simulink model "RR_1DOF"  (R2023b)
settings: Solver=VariableStepAuto  StartTime=0.0  StopTime=1200  RelTol=1e-3
values from neighbouring files (symbols this model uses):
  G = 32.174    [RR.mat]
  RR_AERO_S = 8.85    [RR.mat]
  RR_Fuel_Consumption = [7.65146967075e-05 0.000426716577792]    [RR.mat]
  RR_Fuel_Mass = 0.422701560266    [RR.mat]
  RR_Fuel_Volume = 0.267361092544    [RR.mat]
  RR_Motors_Thrust = [4.04656097579 98.9159349639]    [RR.mat]
  RR_Motors_Thrust_Alt_Lut = [0 10000 20000 30000]    [RR.mat]
  RR_Motors_Thrust_Pct_Lut = [1 0.705882352941 0.470588235294 0.352941176471]    [RR.mat]
  RR_PD_ALT = [0 10000 30000]    [RR.mat]
  RR_PD_CD = [0.03954  0.0426  0.05073; 0.01481  0.01557  0.0175; 0.0113  0.01182  0.01313; 0.0103  0.01077  0.01191]    [RR.mat]
  RR_PD_MACH = [0.001 0.1 0.5 0.9]    [RR.mat]
  RR_Total_Dry_Mass = 1.55129843973    [RR.mat]
undefined symbols (not defined in the file or in its folder): magnitude
libraries: aerolibatmos2 x1, aerolibasang x1, simulink x1
settings Model: Creator=jrighetti  LastModifiedBy=jrighetti

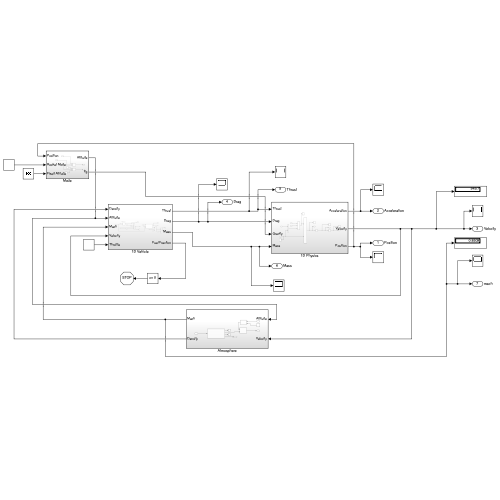
[thumbnail: Simulink's stored preview of the top-level diagram]
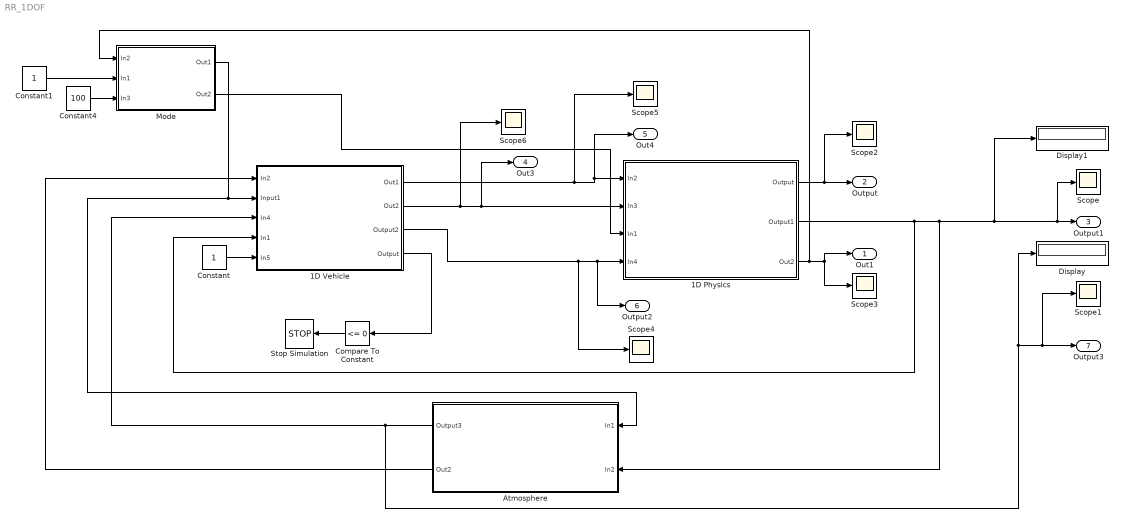
== system RR_1DOF ==
  1D Physics : Subsystem
  1D Vehicle : Subsystem
  Atmosphere : Subsystem
  Compare To Constant : simulink/Logic and Bit Operations/Compare To Constant  relop=<=  const=0  OutDataTypeStr=boolean
  Constant : Constant
  Constant1 : Constant
  Constant4 : Constant  Value=100
  Display : Display
  Display1 : Display
  Mode : Subsystem
  Scope{,1..6} (7 alike) : Scope
  Stop Simulation : Stop
  Out1 : Outport  SignalName=Position
  Output : Outport  Port=2  SignalName=Acceleration
  Output1 : Outport  Port=3  SignalName=Velocity
  Out3 : Outport  Port=4  SignalName=Drag
  Out4 : Outport  Port=5  SignalName=Thrust
  Output2 : Outport  Port=6  SignalName=Mass
  Output3 : Outport  Port=7  SignalName=mach
  wires:
  1D Vehicle/1(Out1) -> Scope5/1, Out4/1, 1D Physics/1(In2)
  1D Vehicle/2(Out2) -> Scope6/1, 1D Physics/2(In3), Out3/1
  1D Vehicle/4(Output) -> Compare To Constant/1
  1D Vehicle/3(Output2) -> Scope4/1, Output2/1, 1D Physics/4(In4)
  Constant/1 -> 1D Vehicle/5(In5)
  Atmosphere/1(Output3) -> Display/1, Scope1/1, Output3/1, 1D Vehicle/3(In4)
  1D Physics/1(Output) -> Scope2/1, Output/1
  1D Physics/3(Out2) -> Mode/1(In2), Out1/1, Scope3/1
  1D Physics/2(Output1) -> Atmosphere/2(In2), Display1/1, Scope/1, Output1/1, 1D Vehicle/4(In1)
  Compare To Constant/1 -> Stop Simulation/1
  Atmosphere/2(Out2) -> 1D Vehicle/1(In2)
  Constant4/1 -> Mode/3(In3)
  Mode/2(Out2) -> 1D Physics/3(In1)
  Constant1/1 -> Mode/2(In1)
  Mode/1(Out1) -> 1D Vehicle/2(Input1), Atmosphere/1(In1)

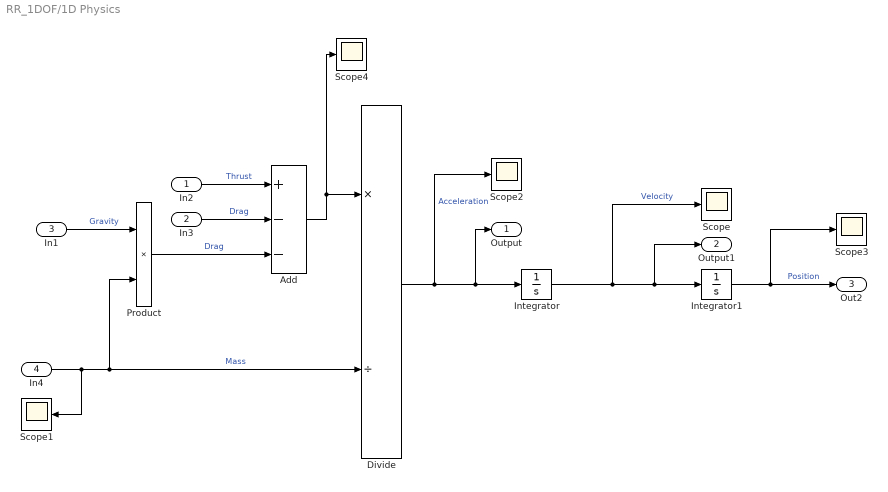
== system RR_1DOF/1D Physics ==
  In2 : Inport
  In3 : Inport  Port=2
  In1 : Inport  Port=3
  In4 : Inport  Port=4
  Add : Sum  Inputs=+--
  Divide : Product  Inputs=*/
  Integrator : Integrator
  Integrator1 : Integrator
  Product : Product
  Scope{,1..4} (5 alike) : Scope
  Output : Outport
  Output1 : Outport  Port=2
  Out2 : Outport  Port=3
  wires:
  Integrator1/1 -> Scope3/1, Out2/1  "Position"
  Add/1 -> Scope4/1, Divide/1
  Integrator/1 -> Integrator1/1, Output1/1, Scope/1  "Velocity"
  Divide/1 -> Scope2/1, Output/1, Integrator/1  "Acceleration"
  In2/1 -> Add/1  "Thrust"
  In3/1 -> Add/2  "Drag"
  In4/1 -> Scope1/1, Divide/2, Product/2  "Mass"
  In1/1 -> Product/1  "Gravity"
  Product/1 -> Add/3  "Drag"

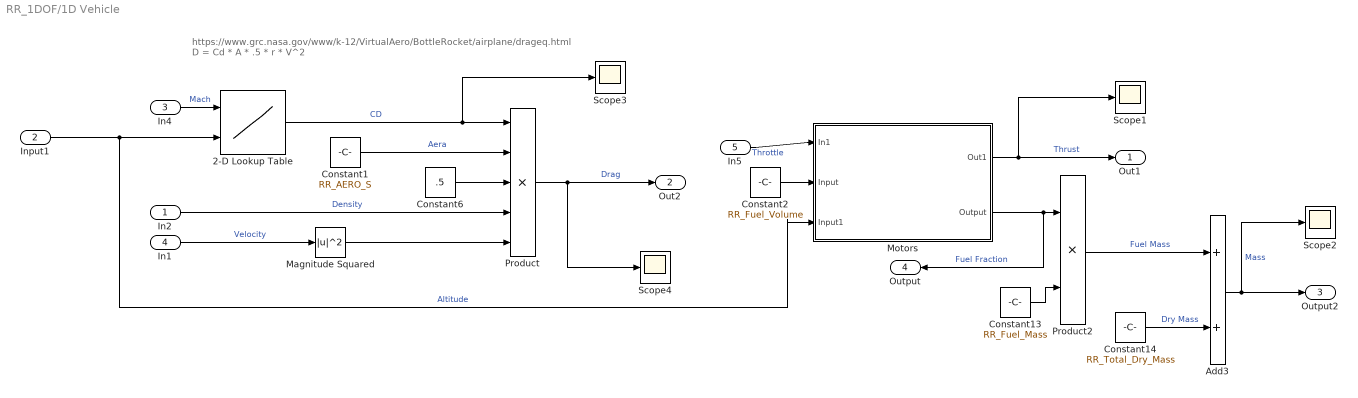
== system RR_1DOF/1D Vehicle ==
  note: https://www.grc.nasa.gov/www/k-12/VirtualAero/BottleRocket/airplane/drageq.html
      |
      | D = Cd * A * .5 * r * V^2
  In2 : Inport
  Input1 : Inport  Port=2
  In4 : Inport  Port=3
  In1 : Inport  Port=4
  In5 : Inport  Port=5
  2-D Lookup Table : Lookup_n-D  BreakpointsForDimension1=RR_PD_MACH  BreakpointsForDimension2=RR_PD_ALT  Table=RR_PD_CD  InternalRulePriority=Speed  RndMeth=Simplest
      settings: InputPortMap=u0,u1
  Add3 : Sum
  Constant1 : Constant  Value=RR_AERO_S
  Constant13 : Constant  Value=RR_Fuel_Mass
  Constant14 : Constant  Value=RR_Total_Dry_Mass
  Constant2 : Constant  Value=RR_Fuel_Volume
  Constant6 : Constant  Value=.5
  Magnitude Squared : Math  Operator=magnitude^2
  Motors : Subsystem
  Product : Product  Inputs=5
  Product2 : Product
  Scope{1..4} (4 alike) : Scope
  Out1 : Outport
  Out2 : Outport  Port=2
  Output2 : Outport  Port=3
  Output : Outport  Port=4
  wires:
  2-D Lookup Table/1 -> Scope3/1, Product/1  "CD"
  Motors/1(Out1) -> Scope1/1, Out1/1  "Thrust"
  Product/1 -> Scope4/1, Out2/1  "Drag"
  Constant1/1 -> Product/2  "Aera"
  Constant6/1 -> Product/3
  In2/1 -> Product/4  "Density"
  Magnitude Squared/1 -> Product/5
  In1/1 -> Magnitude Squared/1  "Velocity"
  Input1/1 -> Motors/3(Input1), 2-D Lookup Table/2  "Altitude"
  In4/1 -> 2-D Lookup Table/1  "Mach"
  Constant2/1 -> Motors/2(Input)
  Constant14/1 -> Add3/2  "Dry Mass"
  Motors/2(Output) -> Product2/1, Output/1  "Fuel Fraction"
  Constant13/1 -> Product2/2
  Product2/1 -> Add3/1  "Fuel Mass"
  Add3/1 -> Scope2/1, Output2/1  "Mass"
  In5/1 -> Motors/1(In1)  "Throttle"

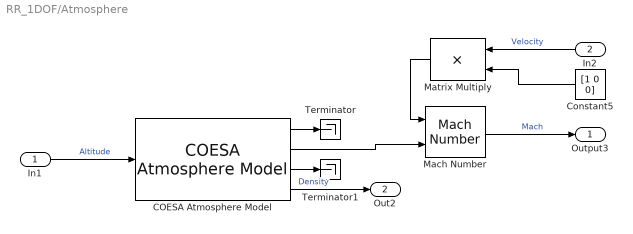
== system RR_1DOF/Atmosphere ==
  In1 : Inport
  In2 : Inport  Port=2
  COESA Atmosphere Model : aerolibatmos2/COESA Atmosphere Model  units=English (Velocity in ft/s)  spec=1976 COESA-extended U.S. Standard Atmosphere  model=Profile  profile_var=High temperature  profile_percent=1%  profile_alt=5 km (16404 ft)  envelope_var=High temperature  envelope_percent=1%  action=Warning
  Constant5 : Constant  Value=[1 0 0]
  Mach Number : aerolibasang/Mach Number
  Matrix Multiply : Product
  Terminator : Terminator
  Terminator1 : Terminator
  Output3 : Outport
  Out2 : Outport  Port=2
  wires:
  COESA Atmosphere Model/3 -> Terminator1/1
  COESA Atmosphere Model/1 -> Terminator/1
  Matrix Multiply/1 -> Mach Number/1
  Constant5/1 -> Matrix Multiply/2
  In2/1 -> Matrix Multiply/1  "Velocity"
  Mach Number/1 -> Output3/1  "Mach"
  COESA Atmosphere Model/2 -> Mach Number/2
  In1/1 -> COESA Atmosphere Model/1  "Altitude"
  COESA Atmosphere Model/4 -> Out2/1  "Density"

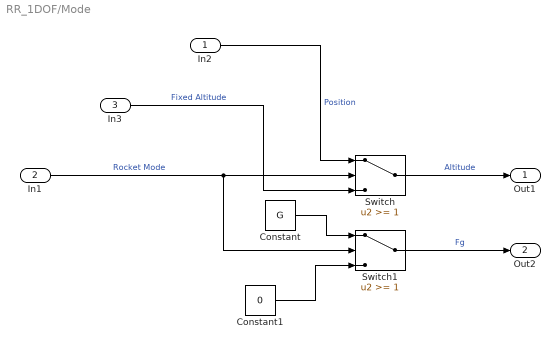
== system RR_1DOF/Mode ==
  In2 : Inport
  In1 : Inport  Port=2
  In3 : Inport  Port=3
  Constant : Constant  Value=G
  Constant1 : Constant  Value=0
  Switch : Switch  Threshold=1  SaturateOnIntegerOverflow=off  InputSameDT=off
  Switch1 : Switch  Threshold=1  SaturateOnIntegerOverflow=off  InputSameDT=off
  Out1 : Outport
  Out2 : Outport  Port=2
  wires:
  In1/1 -> Switch1/2, Switch/2  "Rocket Mode"
  Constant/1 -> Switch1/1
  Constant1/1 -> Switch1/3
  In2/1 -> Switch/1  "Position"
  In3/1 -> Switch/3  "Fixed Altitude"
  Switch/1 -> Out1/1  "Altitude"
  Switch1/1 -> Out2/1  "Fg"

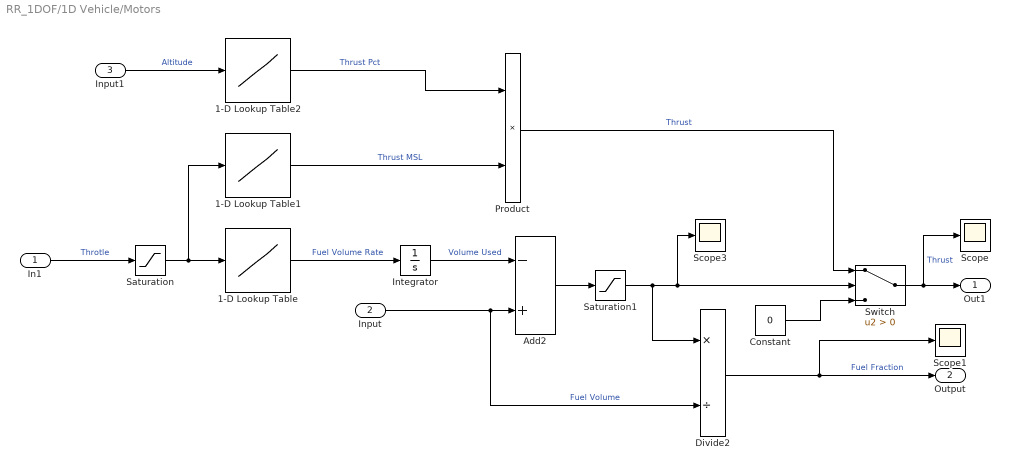
== system RR_1DOF/1D Vehicle/Motors ==
  In1 : Inport
  Input : Inport  Port=2
  Input1 : Inport  Port=3
  1-D Lookup Table : Lookup_n-D  NumberOfTableDimensions=1  BreakpointsForDimension1=[0,1]  Table=RR_Fuel_Consumption  InternalRulePriority=Speed  RndMeth=Simplest
  1-D Lookup Table1 : Lookup_n-D  NumberOfTableDimensions=1  BreakpointsForDimension1=[0,1]  Table=RR_Motors_Thrust  InternalRulePriority=Speed  RndMeth=Simplest
  1-D Lookup Table2 : Lookup_n-D  NumberOfTableDimensions=1  BreakpointsForDimension1=RR_Motors_Thrust_Alt_Lut  Table=RR_Motors_Thrust_Pct_Lut  InternalRulePriority=Speed  RndMeth=Simplest
  Add2 : Sum  Inputs=-+
  Constant : Constant  Value=0
  Divide2 : Product  Inputs=*/
  Integrator : Integrator
  Product : Product
  Saturation : Saturate  UpperLimit=1.0  LowerLimit=0.0
  Saturation1 : Saturate  UpperLimit=10000000  LowerLimit=0
  Scope : Scope
  Scope1 : Scope
  Scope3 : Scope
  Switch : Switch  Criteria=u2 > Threshold  SaturateOnIntegerOverflow=off  InputSameDT=off
  Out1 : Outport
  Output : Outport  Port=2
  wires:
  In1/1 -> Saturation/1  "Throtle"
  Saturation/1 -> 1-D Lookup Table1/1, 1-D Lookup Table/1
  1-D Lookup Table/1 -> Integrator/1  "Fuel Volume Rate"
  Switch/1 -> Scope/1, Out1/1  "Thrust"
  Integrator/1 -> Add2/1  "Volume Used"
  Add2/1 -> Saturation1/1
  Input/1 -> Divide2/2, Add2/2  "Fuel Volume"
  Saturation1/1 -> Scope3/1, Switch/2, Divide2/1
  Constant/1 -> Switch/3
  Divide2/1 -> Scope1/1, Output/1  "Fuel Fraction"
  Input1/1 -> 1-D Lookup Table2/1  "Altitude"
  1-D Lookup Table2/1 -> Product/1  "Thrust Pct"
  1-D Lookup Table1/1 -> Product/2  "Thrust MSL"
  Product/1 -> Switch/1  "Thrust"
